simulink model "system_model"  (R2013a)
settings: Solver=ode45  StartTime=0.0  StopTime=10  RelTol=1e-3
values from neighbouring files (symbols this model uses):
  A = [-.5 .5; 0 -2]    [get_simulation_values.m]
  Ad = dt_sys.a    [get_simulation_values.m]
  B = [0; 2]    [get_simulation_values.m]
  Bd = dt_sys.b    [get_simulation_values.m]
  C = [1 0]    [get_simulation_values.m]
  Kr = -inv( (C-D*K)*inv(Ad-I-Bd*K)*Bd + D )    [get_simulation_values.m]
  L = acker(Ad',C',P_L).'    [get_simulation_values.m]
  Qw = 0    [get_simulation_values.m]
  Rv = 0    [get_simulation_values.m]
undefined symbols (not defined in the file or in its folder): K
settings Model: Creator=Kyle  LastModifiedBy=Kyle

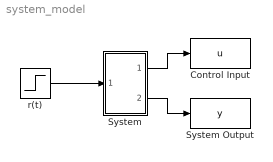
== system system_model ==
  Control Input : ToWorkspace  VariableName=u  SampleTime=-1  SaveFormat=Timeseries
  System : Subsystem  mask{A=A, B=B, C=C, Ad=Ad, Bd=Bd, K=K, Kr=Kr, L=L, Qw=Qw, Rv=Rv}
      mask prompts: A "System Matrix (A)"; B "Output Matrix (B)"; C "Input Matrix (C)"; Ad "Discrete-Time System Matrix (Ad)"; Bd "Discrete-Time Output Matrix (Bd)"; K "Feedback Gains (K)"; Kr "Input Gain (Kr)"; L "Observer Gains (L)"; Qw "Process Noise (Qw)"; Rv "Sensor Noise (Rv)"
  System Output : ToWorkspace  VariableName=y  SampleTime=-1  SaveFormat=Timeseries
  r(t) : Step  Time=0  After=2.5  SampleTime=0
  wires:
  r(t)/1 -> System/1(r[n])
  System/1(u(t)) -> Control Input/1
  System/2(y(t)) -> System Output/1

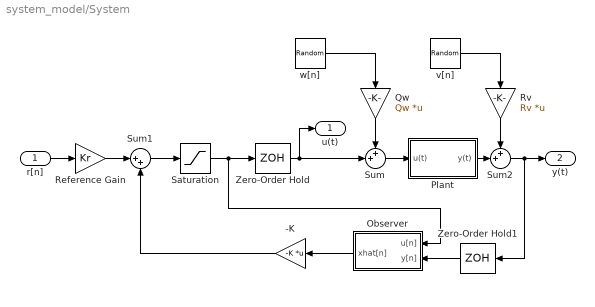
== system system_model/System ==
  r[n] : Inport
  -K : Gain  Gain=-K  Multiplication=Matrix(K*u)
  Observer : Subsystem  mask{Ad=Ad, Bd=Bd, C=C, L=L}
      mask prompts: Ad "System Matrix (Ad)"; Bd "Input Matrix (Bd)"; C "Output Matrix (C)"; L "Observer Gains (L)"
  Plant : Subsystem  mask{A=A, B=B, C=C}
      mask prompts: A "System Matrix (A)"; B "Input Matrix (B)"; C "Output Matrix (C)"
  Qw : Gain  Gain=Qw  Multiplication=Matrix(K*u)
  Reference Gain : Gain  Gain=Kr
  Rv : Gain  Gain=Rv  Multiplication=Matrix(K*u)
  Saturation : Saturate  UpperLimit=5  LowerLimit=0
  Sum : Sum  Inputs=++|
  Sum1 : Sum  Inputs=|++
  Sum2 : Sum  Inputs=++|
  Zero-Order Hold : ZeroOrderHold  SampleTime=0.1
  Zero-Order Hold1 : ZeroOrderHold  SampleTime=0.1
  v[n] : RandomNumber  SampleTime=0.1
  w[n] : RandomNumber  SampleTime=0.1
  u(t) : Outport
  y(t) : Outport  Port=2
  wires:
  Reference Gain/1 -> Sum1/1
  -K/1 -> Sum1/2
  Observer/1(xhat[n]) -> -K/1
  r[n]/1 -> Reference Gain/1
  Zero-Order Hold/1 -> Sum/2, u(t)/1
  Qw/1 -> Sum/1
  w[n]/1 -> Qw/1
  Plant/1(y(t)) -> Sum2/2
  Sum2/1 -> Zero-Order Hold1/1, y(t)/1
  Rv/1 -> Sum2/1
  v[n]/1 -> Rv/1
  Sum1/1 -> Saturation/1
  Saturation/1 -> Observer/1(u[n]), Zero-Order Hold/1
  Zero-Order Hold1/1 -> Observer/2(y[n])
  Sum/1 -> Plant/1(u(t))

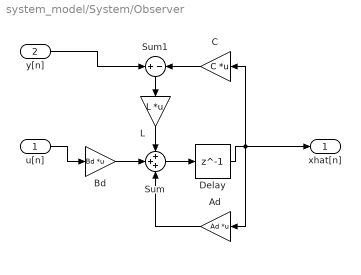
== system system_model/System/Observer ==
  u[n] : Inport
  y[n] : Inport  Port=2
  Ad : Gain  Gain=Ad  Multiplication=Matrix(K*u)
  Bd : Gain  Gain=Bd  Multiplication=Matrix(K*u)
  C : Gain  Gain=C  Multiplication=Matrix(K*u)
  Delay : Delay  DelayLength=1  InitialCondition=0  SampleTime=0.1
  L : Gain  Gain=L  Multiplication=Matrix(K*u)
  Sum : Sum  Inputs=+++
  Sum1 : Sum  Inputs=+|-
  xhat[n] : Outport
  wires:
  C/1 -> Sum1/2
  Ad/1 -> Sum/3
  Sum1/1 -> L/1
  Sum/1 -> Delay/1
  u[n]/1 -> Bd/1
  Delay/1 -> C/1, Ad/1, xhat[n]/1
  L/1 -> Sum/1
  Bd/1 -> Sum/2
  y[n]/1 -> Sum1/1

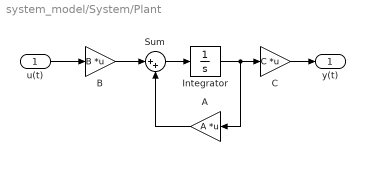
== system system_model/System/Plant ==
  u(t) : Inport
  A : Gain  Gain=A  Multiplication=Matrix(K*u)
  B : Gain  Gain=B  Multiplication=Matrix(K*u)
  C : Gain  Gain=C  Multiplication=Matrix(K*u)
  Integrator : Integrator
  Sum : Sum  Inputs=|++
  y(t) : Outport
  wires:
  u(t)/1 -> B/1
  B/1 -> Sum/1
  A/1 -> Sum/2
  C/1 -> y(t)/1
  Sum/1 -> Integrator/1
  Integrator/1 -> A/1, C/1
